simulink model "proj8_p1"  (R2017a)
settings: Solver=VariableStepAuto  StartTime=0.0  StopTime=10.0  RelTol=1e-3
undefined symbols (not defined in the file or in its folder): mc
settings Model: Creator=admin  LastModifiedBy=admin

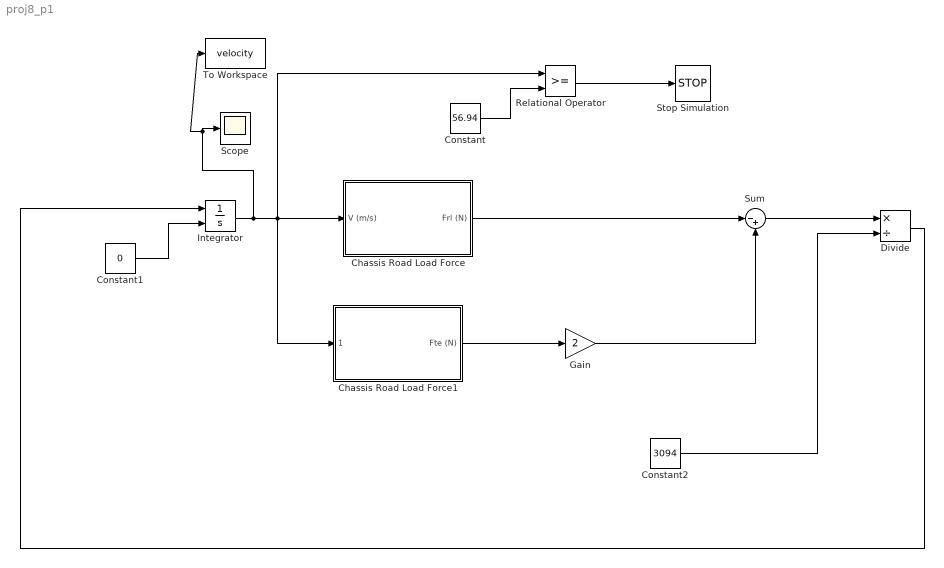
== system proj8_p1 ==
  Chassis Road Load Force : Subsystem  TreatAsAtomicUnit=on
  Chassis Road Load Force1 : Subsystem  TreatAsAtomicUnit=on
  Constant : Constant  Value=56.94
  Constant1 : Constant  Value=0
  Constant2 : Constant  Value=3094
  Divide : Product  Inputs=*/
  Gain : Gain  Gain=2
  Integrator : Integrator  InitialConditionSource=external
  Relational Operator : RelationalOperator  OutDataTypeStr=boolean  RndMeth=Simplest
  Scope : Scope
  Stop Simulation : Stop
  Sum : Sum  Inputs=|-+
  To Workspace : ToWorkspace  VariableName=velocity  SaveFormat=Timeseries  SampleTime=-1
  wires:
  Constant1/1 -> Integrator/2
  Integrator/1 -> To Workspace/1, Scope/1, Chassis Road Load Force1/1(" "), Relational Operator/1, Chassis Road Load Force/1("V (m/s) ")
  Chassis Road Load Force/1(Frl (N)) -> Sum/1
  Chassis Road Load Force1/1(Fte (N)) -> Gain/1
  Sum/1 -> Divide/1
  Constant2/1 -> Divide/2
  Divide/1 -> Integrator/1
  Constant/1 -> Relational Operator/2
  Relational Operator/1 -> Stop Simulation/1
  Gain/1 -> Sum/2

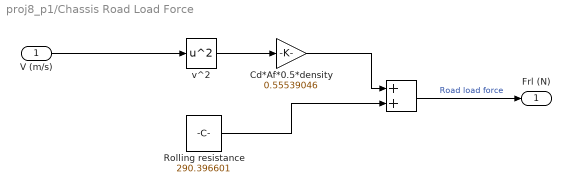
== system proj8_p1/Chassis Road Load Force ==
  "V (m/s) " : Inport
  " " : Sum
  "Cd*Af*0.5*density " : Gain  Gain=0.55539046
  "Rolling resistance " : Constant  Value=290.396601
  v^2 : Math  Operator=square  SaturateOnIntegerOverflow=on
  Frl (N) : Outport
  wires:
  v^2/1 -> "Cd*Af*0.5*density "/1
  "V (m/s) "/1 -> v^2/1
  "Cd*Af*0.5*density "/1 -> " "/1
  "Rolling resistance "/1 -> " "/2
  " "/1 -> Frl (N)/1  "Road load force"

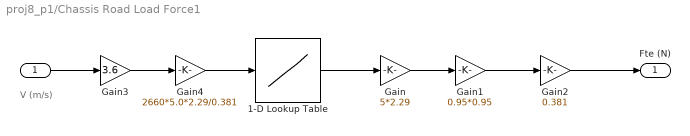
== system proj8_p1/Chassis Road Load Force1 ==
  note: V (m/s)
  " " : Inport
  1-D Lookup Table : Lookup_n-D  NumberOfTableDimensions=1  BreakpointsForDimension1=mc.rpm_max_index  Table=mc.trq_max_map  InternalRulePriority=Speed  RndMeth=Simplest  InputSameDT=on
  Gain : Gain  Gain=5*2.29
  Gain1 : Gain  Gain=0.95*0.95
  Gain2 : Gain  Gain=0.381
  Gain3 : Gain  Gain=3.6
  Gain4 : Gain  Gain=2660*5.0*2.29/0.381
  Fte (N) : Outport
  wires:
  Gain3/1 -> Gain4/1
  " "/1 -> Gain3/1
  Gain4/1 -> 1-D Lookup Table/1
  1-D Lookup Table/1 -> Gain/1
  Gain/1 -> Gain1/1
  Gain1/1 -> Gain2/1
  Gain2/1 -> Fte (N)/1
